simulink model "ExothermicCSTR"  (R2014b)
settings: Solver=ode15s  StartTime=0.0  StopTime=100  MaxStep=0.01  RelTol=1e-3
settings Model: Creator=jeff  LastModifiedBy=jeff

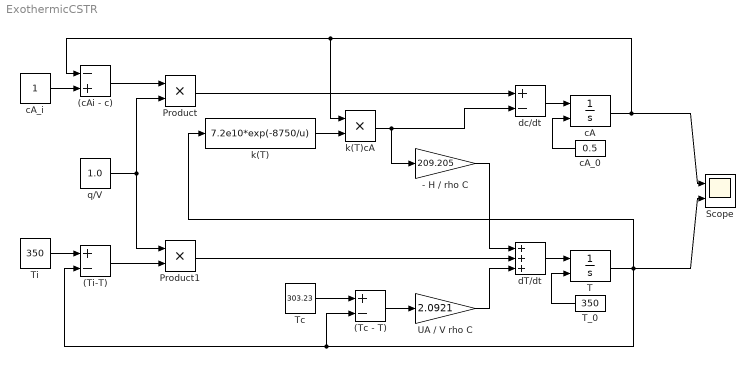
== system ExothermicCSTR ==
  (Tc - T) : Sum  Inputs=+-
  (Ti-T) : Sum  Inputs=+-
  (cAi - c) : Sum  Inputs=-+
  - H / rho C : Gain  Gain=209.205
  Product : Product
  Product1 : Product
  Scope : Scope  NumInputPorts=2
      settings: TimeRange=30  YMin=0~320  YMax=0.9~440
  T : Integrator  InitialConditionSource=external  LimitOutput=on  LowerSaturationLimit=0
  T_0 : Constant  Value=350
  Tc : Constant  Value=303.23
  Ti : Constant  Value=350
  UA / V rho C : Gain  Gain=2.0921
  cA : Integrator  InitialConditionSource=external  LimitOutput=on  LowerSaturationLimit=0
  cA_0 : Constant  Value=0.5
  "cA_i " : Constant
  dT/dt : Sum  Inputs=+++
  dc/dt : Sum  Inputs=+-
  k(T) : Fcn  Expr=7.2e10*exp(-8750/u)
  k(T)cA : Product
  q/V : Constant  Value=1.0
  wires:
  cA/1 -> Scope/1, (cAi - c)/1, k(T)cA/1
  "cA_i "/1 -> (cAi - c)/2
  (cAi - c)/1 -> Product/1
  cA_0/1 -> cA/2
  T_0/1 -> T/2
  T/1 -> k(T)/1, Scope/2, (Ti-T)/2, (Tc - T)/2
  q/V/1 -> Product/2, Product1/1
  (Ti-T)/1 -> Product1/2
  Ti/1 -> (Ti-T)/1
  dc/dt/1 -> cA/1
  Product/1 -> dc/dt/1
  k(T)/1 -> k(T)cA/2
  k(T)cA/1 -> dc/dt/2, - H / rho C/1
  Product1/1 -> dT/dt/2
  dT/dt/1 -> T/1
  - H / rho C/1 -> dT/dt/1
  Tc/1 -> (Tc - T)/1
  UA / V rho C/1 -> dT/dt/3
  (Tc - T)/1 -> UA / V rho C/1
